simulink model "LightManager"  (R2019a)
settings: Solver=FixedStepDiscrete  StartTime=0.0  StopTime=10.0  FixedStep=0.01  RelTol=1e-3  EnableMultiTasking=on
libraries: simulink x2
settings Model: Creator=marsh  LastModifiedBy=marsh
settings DataIOCC: SaveFormat=StructureWithTime
settings OptimizationCC: DefaultParameterBehavior=Inlined  UseDivisionForNetSlopeComputation=on  GainParamInheritBuiltInType=on  UseFloatMulNetSlope=on  InlineInvariantSignals=on  PassReuseOutputArgsAs=Individual arguments  ZeroExternalMemoryAtStartup=off  ZeroInternalMemoryAtStartup=off  NoFixptDivByZeroProtection=on  EfficientFloat2IntCast=on  LifeSpan=1  OptimizeBlockOrder=speed  DifferentSizesBufferReuse=on
settings DebuggingCC: ParameterTunabilityLossMsg=error
settings HardwareCC: ProdBitPerPointer=32  ProdBitPerSizeT=32  ProdBitPerPtrDiffT=32  ProdLargestAtomicInteger=Long  ProdLargestAtomicFloat=Double  ProdWordSize=32  ProdLongLongMode=on  ProdHWDeviceType=NXP->Cortex-M4
settings ModelReferenceCC: ModelReferenceNumInstancesAllowed=Single
settings SFSimCC: MATLABDynamicMemAlloc=off
settings RTWCC: SystemTargetFile=autosar.tlc  GenCodeOnly=on  TemplateMakefile=ert_default_tmf  Description=AUTOSAR  GenerateReport=on  IncludeHyperlinkInReport=on  LaunchReport=on  GenerateTraceInfo=on  GenerateTraceReport=on  GenerateTraceReportSl=on  GenerateTraceReportSf=on  GenerateTraceReportEml=on  GenerateCodeMetricsReport=on
settings CodeAppCC: ForceParamTrailComments=on  IgnoreCustomStorageClasses=off  OperatorAnnotations=on  SimulinkDataObjDesc=on  SFDataObjDesc=on  CustomSymbolStrGlobalVar=rt$N$M  CustomSymbolStrType=$N$M  CustomSymbolStrFcn=$N$M$F  CustomSymbolStrMacro=$N$M  InsertBlockDesc=on
settings STFCustomTargetCC: TargetLangStandard=C99 (ISO)  MultiwordLength=256  ParMdlRefBuildCompliant=on  CompOptLevelCompliant=on  IncludeMdlTerminateFcn=off  CombineOutputUpdateFcns=on  CombineSignalStateStructs=on  SuppressErrorStatus=on  ERTCustomFileBanners=on  SupportAbsoluteTime=off  SupportNonFinite=off  SupportComplex=off  SupportContinuousTime=off  SupportNonInlinedSFcns=off  RemoveResetFunc=on  MATLABClassNameForMDSCustomization=Simulink.SoftwareTarget.ERTCustomization  AutosarCompliant=on  GRTInterface=off  UseToolchainInfoCompliant=on  LookupTableObjectStructAxisOrder=2,1,3,4,...  LUTObjectStructOrderEvenSpacing=Size,Table,Breakpoints  SystemTargetFile=autosar.tlc
settings ERTTargetCC: TargetLangStandard=C99 (ISO)  ConcurrentExecutionCompliant=off  IncludeMdlTerminateFcn=off  CombineSignalStateStructs=on  SuppressErrorStatus=on  SupportAbsoluteTime=off  SupportNonFinite=off  SupportComplex=off  ModelStepFunctionPrototypeControlCompliant=off  CPPClassGenCompliant=off  AutosarCompliant=on  LookupTableObjectStructAxisOrder=2,1,3,4,...  LUTObjectStructOrderEvenSpacing=Size,Table,Breakpoints  InlinedParameterPlacement=NonHierarchical  ERTCustomFileTemplate=example_file_process.tlc  ERTFilePackagingFormat=CompactWithDataFile

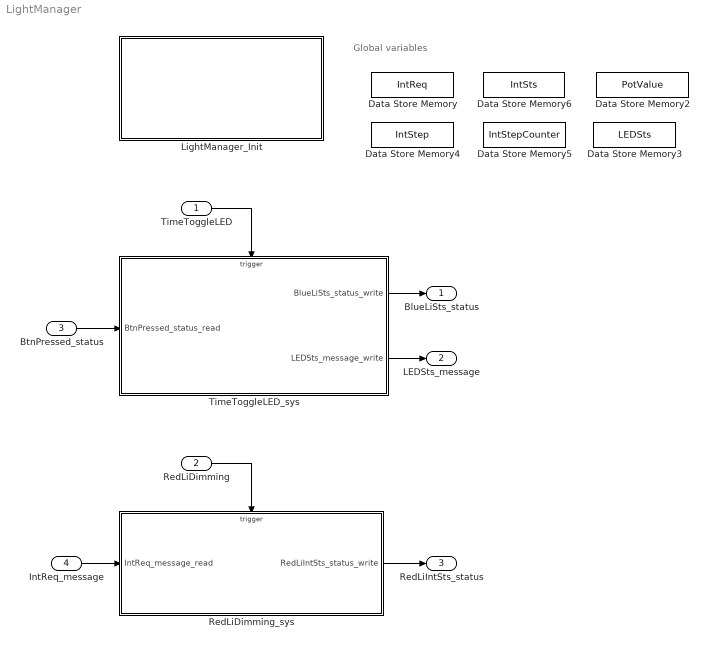
== system LightManager ==
  note: Global variables
  TimeToggleLED : Inport  SampleTime=0.01  OutputFunctionCall=on
  RedLiDimming : Inport  Port=2  SampleTime=0.01  OutputFunctionCall=on
  BtnPressed_status : Inport  Port=3  OutDataTypeStr=SwitchStatus  PortDimensions=1
  IntReq_message : Inport  Port=4  OutDataTypeStr=Int  PortDimensions=1
  Data Store Memory : DataStoreMemory  DataStoreName=IntReq  ReadBeforeWriteMsg=warning  WriteAfterWriteMsg=warning  WriteAfterReadMsg=warning  ShowAdditionalParam=off  OutDataTypeStr=uint8
  Data Store Memory2 : DataStoreMemory  DataStoreName=PotValue  ReadBeforeWriteMsg=warning  WriteAfterWriteMsg=warning  WriteAfterReadMsg=warning  InitialValue=0.1  ShowAdditionalParam=off  OutMin=[0.1]  OutMax=[2.65]  OutDataTypeStr=uint8
  Data Store Memory3 : DataStoreMemory  DataStoreName=LEDSts  ReadBeforeWriteMsg=warning  WriteAfterWriteMsg=warning  WriteAfterReadMsg=warning  InitialValue=1  ShowAdditionalParam=off  OutDataTypeStr=boolean
  Data Store Memory4 : DataStoreMemory  DataStoreName=IntStep  ReadBeforeWriteMsg=warning  WriteAfterWriteMsg=warning  WriteAfterReadMsg=warning  ShowAdditionalParam=off  OutDataTypeStr=double
  Data Store Memory5 : DataStoreMemory  DataStoreName=IntStepCounter  ReadBeforeWriteMsg=warning  WriteAfterWriteMsg=warning  WriteAfterReadMsg=warning  ShowAdditionalParam=off  OutDataTypeStr=uint8
  Data Store Memory6 : DataStoreMemory  DataStoreName=IntSts  ReadBeforeWriteMsg=warning  WriteAfterWriteMsg=warning  WriteAfterReadMsg=warning  ShowAdditionalParam=off  OutDataTypeStr=double
  LightManager_Init : Subsystem
  RedLiDimming_sys : Subsystem
  TimeToggleLED_sys : Subsystem
  BlueLiSts_status : Outport  OutDataTypeStr=LEDStatus  PortDimensions=1
  LEDSts_message : Outport  Port=2  OutDataTypeStr=Int  PortDimensions=1
  RedLiIntSts_status : Outport  Port=3  OutDataTypeStr=IntensityStatus  PortDimensions=1
  wires:
  BtnPressed_status/1 -> TimeToggleLED_sys/1(BtnPressed_status_read)
  TimeToggleLED_sys/1(BlueLiSts_status_write) -> BlueLiSts_status/1
  TimeToggleLED_sys/2(LEDSts_message_write) -> LEDSts_message/1
  IntReq_message/1 -> RedLiDimming_sys/1(IntReq_message_read)
  RedLiDimming_sys/1(RedLiIntSts_status_write) -> RedLiIntSts_status/1
  TimeToggleLED/1 -> TimeToggleLED_sys/Trigger
  RedLiDimming/1 -> RedLiDimming_sys/Trigger

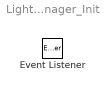
== system LightManager/LightManager_Init ==
  Event Listener : EventListener  EventName=reset

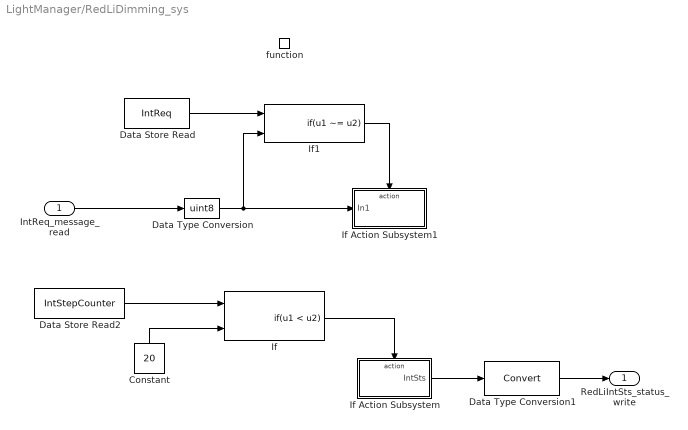
== system LightManager/RedLiDimming_sys ==
  IntReq_message_read : Inport
  function : TriggerPort  TriggerType=function-call  VariantControl=(inherit)  SampleTimeType=periodic  SampleTime=-1
  Constant : Constant  Value=20  OutDataTypeStr=uint8
  Data Store Read : DataStoreRead  DataStoreName=IntReq
  Data Store Read2 : DataStoreRead  DataStoreName=IntStepCounter
  Data Type Conversion : DataTypeConversion  OutDataTypeStr=uint8
  Data Type Conversion1 : DataTypeConversion
  If : If  NumInputs=2  IfExpression=u1 < u2  ShowElse=off
  If Action Subsystem : Subsystem  TreatAsAtomicUnit=on
  If Action Subsystem1 : Subsystem  TreatAsAtomicUnit=on
  If1 : If  NumInputs=2  IfExpression=u1 ~= u2  ShowElse=off
  RedLiIntSts_status_write : Outport
      settings: EnsureOutportIsVirtual=on
  wires:
  Data Store Read2/1 -> If/1
  Constant/1 -> If/2
  If/1 -> If Action Subsystem/Action
  Data Type Conversion/1 -> If1/2, If Action Subsystem1/1(In1)
  Data Store Read/1 -> If1/1
  If1/1 -> If Action Subsystem1/Action
  IntReq_message_read/1 -> Data Type Conversion/1
  Data Type Conversion1/1 -> RedLiIntSts_status_write/1
  If Action Subsystem/1(IntSts) -> Data Type Conversion1/1

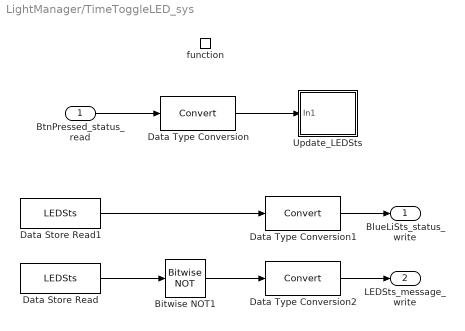
== system LightManager/TimeToggleLED_sys ==
  BtnPressed_status_read : Inport
  function : TriggerPort  TriggerType=function-call  VariantControl=(inherit)  SampleTimeType=periodic  SampleTime=-1
  Bitwise NOT1 : simulink/Logic and Bit Operations/Bitwise Operator  logicop=NOT  UseBitMask=off  BitMask=bin2dec('11011001')  BitMaskRealWorld=Stored Integer
  Data Store Read : DataStoreRead  DataStoreName=LEDSts
  Data Store Read1 : DataStoreRead  DataStoreName=LEDSts
  Data Type Conversion : DataTypeConversion
  Data Type Conversion1 : DataTypeConversion
  Data Type Conversion2 : DataTypeConversion
  Update_LEDSts : Subsystem
  BlueLiSts_status_write : Outport
      settings: EnsureOutportIsVirtual=on
  LEDSts_message_write : Outport  Port=2
      settings: EnsureOutportIsVirtual=on
  wires:
  BtnPressed_status_read/1 -> Data Type Conversion/1
  Data Type Conversion1/1 -> BlueLiSts_status_write/1
  Data Type Conversion2/1 -> LEDSts_message_write/1
  Data Store Read/1 -> Bitwise NOT1/1
  Data Type Conversion/1 -> Update_LEDSts/1(In1)
  Data Store Read1/1 -> Data Type Conversion1/1
  Bitwise NOT1/1 -> Data Type Conversion2/1

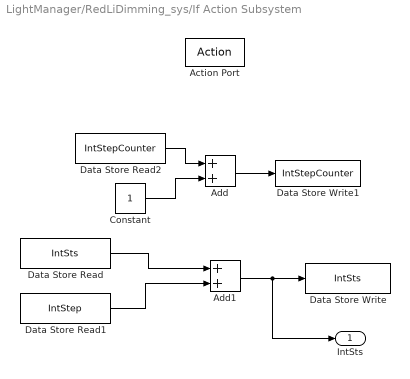
== system LightManager/RedLiDimming_sys/If Action Subsystem ==
  Action Port : ActionPort  ActionPortLabel=if(u1 < u2)
  Add : Sum
  Add1 : Sum
  Constant : Constant  OutDataTypeStr=uint8
  Data Store Read : DataStoreRead  DataStoreName=IntSts
  Data Store Read1 : DataStoreRead  DataStoreName=IntStep
  Data Store Read2 : DataStoreRead  DataStoreName=IntStepCounter
  Data Store Write : DataStoreWrite  DataStoreName=IntSts
  Data Store Write1 : DataStoreWrite  DataStoreName=IntStepCounter
  IntSts : Outport
  wires:
  Constant/1 -> Add/2
  Add/1 -> Data Store Write1/1
  Data Store Read1/1 -> Add1/2
  Add1/1 -> IntSts/1, Data Store Write/1
  Data Store Read2/1 -> Add/1
  Data Store Read/1 -> Add1/1

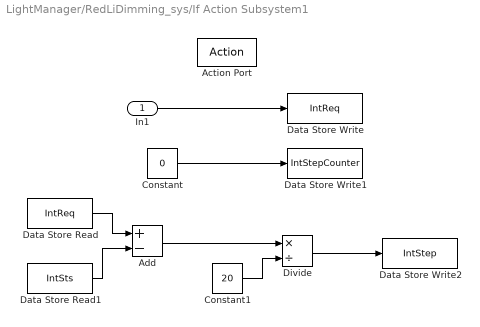
== system LightManager/RedLiDimming_sys/If Action Subsystem1 ==
  In1 : Inport
  Action Port : ActionPort  ActionPortLabel=if(u1 ~= u2)
  Add : Sum  Inputs=+-
  Constant : Constant  Value=0  OutDataTypeStr=uint8
  Constant1 : Constant  Value=20
  Data Store Read : DataStoreRead  DataStoreName=IntReq
  Data Store Read1 : DataStoreRead  DataStoreName=IntSts
  Data Store Write : DataStoreWrite  DataStoreName=IntReq
  Data Store Write1 : DataStoreWrite  DataStoreName=IntStepCounter
  Data Store Write2 : DataStoreWrite  DataStoreName=IntStep
  Divide : Product  Inputs=*/
  wires:
  In1/1 -> Data Store Write/1
  Constant/1 -> Data Store Write1/1
  Data Store Read/1 -> Add/1
  Data Store Read1/1 -> Add/2
  Add/1 -> Divide/1
  Constant1/1 -> Divide/2
  Divide/1 -> Data Store Write2/1

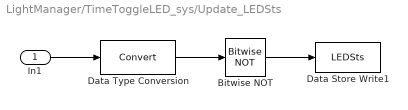
== system LightManager/TimeToggleLED_sys/Update_LEDSts ==
  In1 : Inport
  Bitwise NOT : simulink/Logic and Bit Operations/Bitwise Operator  logicop=NOT  UseBitMask=off  BitMask=bin2dec('11011001')  BitMaskRealWorld=Stored Integer
  Data Store Write1 : DataStoreWrite  DataStoreName=LEDSts
  Data Type Conversion : DataTypeConversion
  wires:
  Data Type Conversion/1 -> Bitwise NOT/1
  In1/1 -> Data Type Conversion/1
  Bitwise NOT/1 -> Data Store Write1/1
